simulink model "model"  (R2015a)
settings: Solver=ode45  StartTime=0.0  StopTime=50  RelTol=1e-3
values from neighbouring files (symbols this model uses):
  Ap = [-R/L,0,0; 0,0,1; 1/L, -Kh/M, -Ch/M]    [script.m]
  Bp = [1;0;0]    [script.m]
  Cp = [0,-10^5/M,0]    [script.m]
  Dp = 0    [script.m]
  Gamma = 1+1e-01    (= 1.1)    [script.m]
  Ki = -0.19405    [script.m]
  Kx = place(A,B,[-60, -50,-40])    [script.m]
  L = 0.0220    (= 0.022)    [script.m]
  Lx = place(Ap',Cp',[-600,-500,-400])'    [script.m]
  M = 1.35    [script.m]
  Theta = [10,10,10,10,10,10]    [script.m]
undefined symbols (not defined in the file or in its folder): A, B, C
settings Model: Creator=jinkale  LastModifiedBy=jinkale

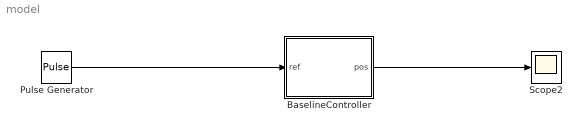
== system model ==
  BaselineController : Subsystem
  Pulse Generator : DiscretePulseGenerator  PulseType=Time based  Period=10  PulseWidth=50  PhaseDelay=10
  Scope2 : Scope
      settings: SaveName=ScopeData2
  wires:
  Pulse Generator/1 -> BaselineController/1(ref)
  BaselineController/1(pos) -> Scope2/1

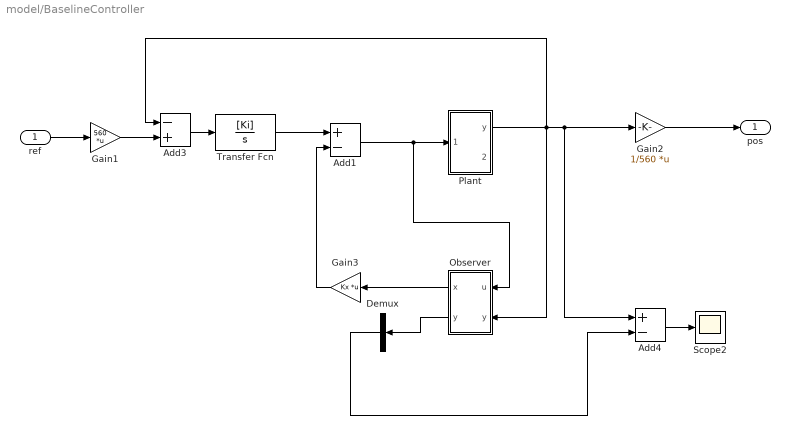
== system model/BaselineController ==
  ref : Inport
  Add1 : Sum  Inputs=+-
  Add3 : Sum  Inputs=-+
  Add4 : Sum  Inputs=+-
  Demux : Demux  Outputs=3
  Gain1 : Gain  Gain=560  Multiplication=Matrix(K*u) (u vector)
  Gain2 : Gain  Gain=1/560  Multiplication=Matrix(K*u) (u vector)
  Gain3 : Gain  Gain=Kx  Multiplication=Matrix(K*u)
  Observer : Subsystem
  Plant : Subsystem
  Scope2 : Scope
      settings: SaveName=ScopeData5
  Transfer Fcn : TransferFcn  Numerator=[Ki]  Denominator=[1 0]
  pos : Outport
  wires:
  Transfer Fcn/1 -> Add1/1
  Add3/1 -> Transfer Fcn/1
  Observer/2("y ") -> Demux/1
  Plant/1(y) -> Observer/2(y), Add4/1, Gain2/1, Add3/1
  Add1/1 -> Observer/1(u), Plant/1(In1)
  Demux/2 -> Add4/2
  Gain3/1 -> Add1/2
  ref/1 -> Gain1/1
  Observer/1("x ") -> Gain3/1
  Add4/1 -> Scope2/1
  Gain2/1 -> pos/1
  Gain1/1 -> Add3/2

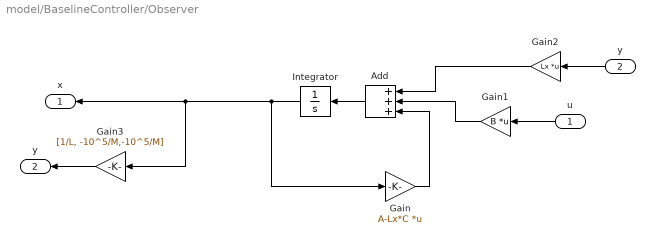
== system model/BaselineController/Observer ==
  u : Inport
  y : Inport  Port=2
  Add : Sum  Inputs=+++
  Gain : Gain  Gain=A-Lx*C  Multiplication=Matrix(K*u)
  Gain1 : Gain  Gain=B  Multiplication=Matrix(K*u)
  Gain2 : Gain  Gain=Lx  Multiplication=Matrix(K*u)
  Gain3 : Gain  Gain=[1/L, -10^5/M,-10^5/M]
  Integrator : Integrator
  "x " : Outport
  "y " : Outport  Port=2
  wires:
  Add/1 -> Integrator/1
  Integrator/1 -> Gain/1, Gain3/1, "x "/1
  Gain/1 -> Add/3
  Gain1/1 -> Add/2
  Gain2/1 -> Add/1
  y/1 -> Gain2/1
  u/1 -> Gain1/1
  Gain3/1 -> "y "/1

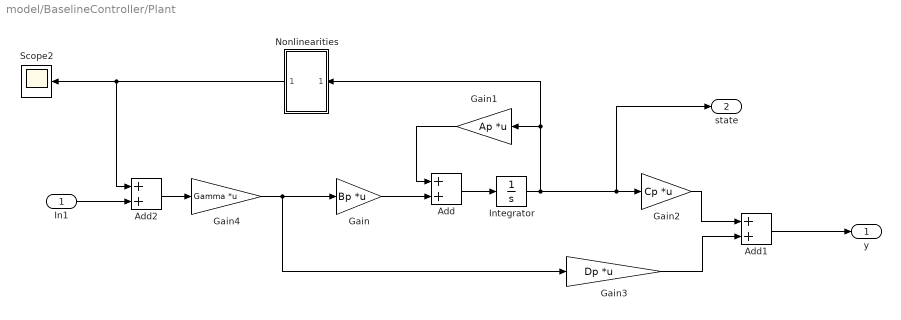
== system model/BaselineController/Plant ==
  In1 : Inport
  Add : Sum
  Add1 : Sum
  Add2 : Sum
  Gain : Gain  Gain=Bp  Multiplication=Matrix(K*u)
  Gain1 : Gain  Gain=Ap  Multiplication=Matrix(K*u)
  Gain2 : Gain  Gain=Cp  Multiplication=Matrix(K*u)
  Gain3 : Gain  Gain=Dp  Multiplication=Matrix(K*u)
  Gain4 : Gain  Gain=Gamma  Multiplication=Matrix(K*u)
  Integrator : Integrator
  Nonlinearities : Subsystem
  Scope2 : Scope
  y : Outport
  state : Outport  Port=2
  wires:
  Gain/1 -> Add/2
  Add/1 -> Integrator/1
  Integrator/1 -> state/1, Gain2/1, Nonlinearities/1(state), Gain1/1
  Gain1/1 -> Add/1
  Gain2/1 -> Add1/1
  Gain3/1 -> Add1/2
  Add1/1 -> y/1
  Gain4/1 -> Gain3/1, Gain/1
  In1/1 -> Add2/2
  Add2/1 -> Gain4/1
  Nonlinearities/1(out) -> Add2/1, Scope2/1

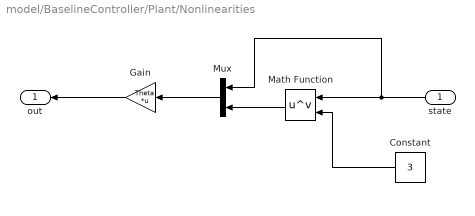
== system model/BaselineController/Plant/Nonlinearities ==
  state : Inport
  Constant : Constant  Value=3
  Gain : Gain  Gain=Theta  Multiplication=Matrix(K*u)
  Math Function : Math  Operator=pow  SaturateOnIntegerOverflow=on
  Mux : Mux  Inputs=2
  out : Outport
  wires:
  state/1 -> Mux/1, Math Function/1
  Constant/1 -> Math Function/2
  Math Function/1 -> Mux/2
  Mux/1 -> Gain/1
  Gain/1 -> out/1
